simulink model "XMC_FFT2D_HLS_AIE"  (R2021a)
settings: Solver=VariableStepAuto  StartTime=0.0  StopTime=256*256*2  RelTol=1e-3
PreLoadFcn:
  | % display k space image & load arrays for
  | % simulation run
  | MRIDemo_PreloadFcn;
undefined symbols (not defined in the file): gray, S, vsva2197, xcvc1902
libraries: dspxfrm3 x2, dspsrcs4 x2, aieDSP x2, simulink x1, vmcUtilities x1, aieUtilities x1, hlsBasic x1
settings Model: Creator=mmi  LastModifiedBy=abehbood
settings SolverCC: AlgebraicLoopSolver=TrustRegion
settings DataIOCC: ReturnWorkspaceOutputs=off
settings DebuggingCC: SFMachineParentedDataDiag=warning  ArithmeticOperatorsInVariantConditions=warning
settings SFSimCC: SimUseLocalCustomCode=off  CustomCodeUndefinedFunction=UseInterfaceOnly
settings RTWCC: RTWUseLocalCustomCode=off

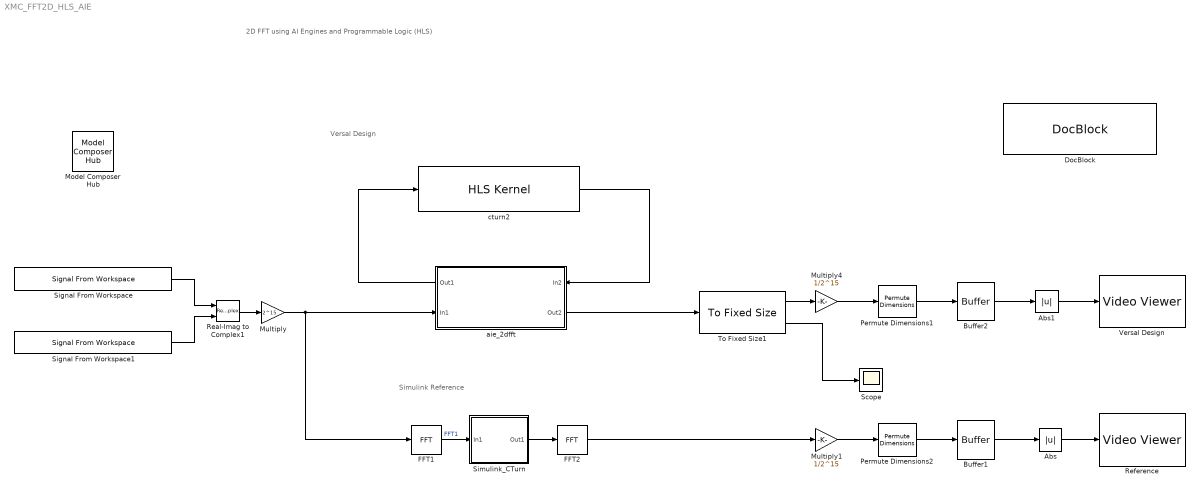
== system XMC_FFT2D_HLS_AIE ==
  note: Versal Design
  note: Simulink Reference
  note: 2D FFT using
      | AI Engines and Programmable Logic (HLS)
  Abs : Abs
  Abs1 : Abs
  Buffer1 : Buffer  N=256  OutputFrames=off
  Buffer2 : Buffer  N=256  OutputFrames=off
  DocBlock : simulink/Model-Wide Utilities/DocBlock  DocumentType=Text  mask(DocBlock){}
      content=|
      | ///////////////////////////////////////////////////////////////////////////
      | // Copyright 2021 Xilinx
      | //
      | // Licensed under the Apache License, Version 2.0 (the "License");
      | // you may not use this file except in compliance with the License.
      | // You may obtain a copy of the License at
      | //
      | // http://www.apache.org/licenses/LICENSE-2.0
      | //
      | // Unless required by applicable law or agreed to in writing, software
      | // distributed under the License is distributed on an "AS IS" BASIS,
      | // WITHOUT WARRANTIES OR CONDITIONS OF ANY KIND, either express or implied.
      | // See the License for the specific language governing permissions and
      | // limitations under the License.
      | ///////////////////////////////////////////////////////////////////////////
      mask Display:
      | xmcDrawBlockIcon();
      | disp(['{\fontsize{10pt}(c) Copyright 2021' ' Xilinx, Inc.}\newline \newline '],'texmode','on');
      | disp('{\fontsize{10pt}Licensed under the Apache License 2.0}','texmode','on');
      | disp('\newline \newline \newline{\fontsize{10pt}Double Click for Copyright Notice}','texmode','on');
  FFT1 : dspxfrm3/FFT  FFTImplementation=Auto  CompMethod=Table lookup  TableOpt=NEW  TableOptActive=Speed  BitRevOrder=off  Normalize=off  InheritFFTLength=on  FFTLength=64  WrapInput=on  roundingMode=Floor  overflowMode=off  firstCoeffDataTypeStr=Inherit: Same word length as input  firstCoeffLastDataTypeStr=Inherit: Same word length as input  prodOutputMode=Binary point scaling  prodOutputWordLength=32  prodOutputFracLength=0  prodOutputDataTypeStr=fixdt(1,32,0)  prodOutputLastDataTypeStr=fixdt(1,32,0)  accumMode=Binary point scaling  accumWordLength=48  accumFracLength=0  accumDataTypeStr=fixdt(1,48,0)  accumLastDataTypeStr=fixdt(1,48,0)  outputMode=Binary point scaling  outputWordLength=16  outputFracLength=0  outputDataTypeStr=fixdt(1,16,0)  outputMin=[]  outputMax=[]  outputLastDataTypeStr=fixdt(1,16,0)
  FFT2 : dspxfrm3/FFT  FFTImplementation=Auto  CompMethod=Table lookup  TableOpt=NEW  TableOptActive=Speed  BitRevOrder=off  Normalize=off  InheritFFTLength=on  FFTLength=64  WrapInput=on  roundingMode=Floor  overflowMode=off  firstCoeffDataTypeStr=Inherit: Same word length as input  firstCoeffLastDataTypeStr=Inherit: Same word length as input  prodOutputMode=Binary point scaling  prodOutputWordLength=32  prodOutputFracLength=0  prodOutputDataTypeStr=fixdt(1,32,0)  prodOutputLastDataTypeStr=fixdt(1,32,0)  accumMode=Binary point scaling  accumWordLength=48  accumFracLength=0  accumDataTypeStr=fixdt(1,48,0)  accumLastDataTypeStr=fixdt(1,48,0)  outputMode=Binary point scaling  outputWordLength=16  outputFracLength=0  outputDataTypeStr=fixdt(1,16,0)  outputMin=[]  outputMax=[]  outputLastDataTypeStr=fixdt(1,16,0)
  Model Composer Hub : vmcUtilities/Model Composer Hub  Tag=genX  CodeGeneration=off  SubsystemName=aie_2dfft  TargetDirectory=./code_fft_graph  ExportType=AI Engines  IpVendor=xilinx.com  IpLibrary=hls  IpVersion=1.0  IpHWLanguage=Verilog  AieCompilerOptions={}  CreateTestbench=on  TestbenchStackSize=10  RunAieSim=on  AieSimTimeout=50000  RunAieSimProfiling=off  LaunchVitisAnalyzer=off  PlotOutput=off  RunX86Sim=off  X86SimTimeout=10  GenHwImage=off  PlatformType=Not Specified  HwSystemType=Baremetal  HwValidationTarget=hw  ProjDevice=xcvc1902-vsva2197-2MP-e-S  ProjDevicePart=xcvc1902-vsva2197-2MP-e-S  SamplePeriod=-1  ClockFrequency=200  DataPathParallelism=1  xilinxfamily=Kintex7  part=xc7k325t  speed=-3  package=fbg676  directory=./netlist  testbench=off  incr_netlist=off  synthesis_tool=Vivado  clock_wrapper=Clock Enables  dbl_ovrd=According to Block Masks  dcm_input_clock_period=10  sysclk_period=10  simulink_period=1  eval_field=0
  Multiply : Gain  Gain=2^15  OutDataTypeStr=int16
  Multiply1 : Gain  Gain=1/2^15  OutDataTypeStr=single
  Multiply4 : Gain  Gain=1/2^15  OutDataTypeStr=single
  Permute Dimensions1 : PermuteDimensions
  Permute Dimensions2 : PermuteDimensions
  Real-Imag to Complex1 : RealImagToComplex
  Reference : VideoViewer  Description=Simulink MRI Display  colormapValue=gray(256)  FigPos=[146 769 633 291]
  Scope : Scope
  Signal From Workspace : dspsrcs4/Signal From Workspace  X=MRIDemo_data_real_channel  Ts=1  nsamps=256  OutputAfterFinalValue=Setting to zero  ignoreOrWarnInputAndFrameLengths=off  OutputFrames=off
  Signal From Workspace1 : dspsrcs4/Signal From Workspace  X=MRIDemo_data_imag_channel  Ts=1  nsamps=256  OutputAfterFinalValue=Setting to zero  ignoreOrWarnInputAndFrameLengths=off  OutputFrames=off
  Simulink_CTurn : Subsystem
  To Fixed Size1 : aieUtilities/To Fixed Size  OutputSize=256  CopyMethod=Buffer samples to form output  HasStatusOutput=off
  Versal Design : VideoViewer  Description=Simulink MRI Display  colormapValue=gray(256)  FigPos=[1240 884 685 270]
  aie_2dfft : Subsystem
      settings: PortSchema="{\"entries\":[{\"content\":{\"sides\":[{\"content\":{\"connectorIds\":[\"Out2\",\"In1\"]},\"type\":\"ConnectorPlacement.EquallySpacedRectSide\",\"uuid\":\"79f05cc3-f11a-4cde-8fa1-dcc9430b22c8\"},{\"content\":{\"connectorIds\":[\"In2\",\"Out1\"],\"side\":\"RIGHT\"},\"type\":\"ConnectorPlacement.EquallySpacedRectSide\",\"uuid\":\"dca5e86a-9095-4cba-ba8f-7e749e0dbd7e\"},{\"content\":{\"connectorIds\":[],\"side\":\"TOP\"},\"type\":\"ConnectorPlacement.EquallySpacedRectSide\",\"uuid\":\"3830c194-8485-43cd-afe1-c92005d5a3f9\"}]},\"type\":\"ConnectorPlacement.EquallySpacedConnector\",\"uuid\":\"40ec3e32-3e8f-4730-8170-0d4e5db1f984\"}],\"packageUris\":[\"http://schema.mathworks.com/mf0/Connector/19700101\"],\"version\":\"1.0\"}"
  cturn2 : hlsBasic/HLS Kernel  PortNames={}  PortSerializedTypes={}  FunctionTemplateParamNames={}  FunctionTemplateParamKinds={}  FunctionTemplateParamTypes={}  FunctionTemplateParamValues={}  PortSynchronicities={'auto'; 'auto'}  PortSignalSizes={0.000000000000000000e+00; 2.560000000000000000e+02}  FunctionTemplateParams={}  FunctionTemplateParamsEnables={}  FunctionTemplateParamsVisible=off  FunctionDeclTypeOptions=C[1 1]@t7@<empty>  PortAttributesTable={ 'Input', 'vin', 'hls::stream< std::complex< int16 >, 0 > &', '', ''; 'Output', 'vout', 'hls::stream< std::complex< int16 >, 0 > &', '', '256' }  PortAttributesEnablement={'off', 'off', 'off', 'off', 'off';'off', 'off', 'off', 'off', 'on'}  SampleTime=-1  PortDirectionTable={ 'vin', 'hls::stream< std::complex< int16 >, 0 > &', 'Input'; 'vout', 'hls::stream< std::complex< int16 >, 0 > &', 'Output' }  PortDirectionTabVisible=on  ArgDirections={1.000000000000000000e+00; 2.000000000000000000e+00}  FunctionIndex=1  FormalArgDecls={'hls::stream< std::complex< int16 >, 0 > & vin', 'hls::stream< std::complex< int16 >, 0 > & vout'}  SimLibPath=''  FunctionTabVisible=on  FunctionDescription=void cturn2(hls::stream< std::complex< int16 >, 0 > & vin, hls::stream< std::complex< int16 >, 0 > & vout)  KernelHeaderFile=./src/cturn2.h  KernelFunction=cturn2  KernelFunctionSelect=<empty>  KernelSourceFile=./src/cturn2.cpp  KernelSearchPaths={}  PreProcOptions={}  blockJsonConstraints=[]  deprecateConstraints=0
  wires:
  Signal From Workspace/1 -> Real-Imag to Complex1/1
  Signal From Workspace1/1 -> Real-Imag to Complex1/2
  FFT2/1 -> Multiply1/1
  Buffer1/1 -> Abs/1
  Permute Dimensions2/1 -> Buffer1/1
  Abs/1 -> Reference/1
  FFT1/1 -> Simulink_CTurn/1(In1)  "FFT1"
  Simulink_CTurn/1(Out1) -> FFT2/1
  Multiply/1 -> FFT1/1, aie_2dfft/1(In1)
  Multiply1/1 -> Permute Dimensions2/1
  Real-Imag to Complex1/1 -> Multiply/1
  Buffer2/1 -> Abs1/1
  Abs1/1 -> Versal Design/1
  To Fixed Size1/1 -> Multiply4/1
  Permute Dimensions1/1 -> Buffer2/1
  aie_2dfft/1(Out2) -> To Fixed Size1/1
  Multiply4/1 -> Permute Dimensions1/1
  aie_2dfft/2(Out1) -> cturn2/1
  cturn2/1 -> aie_2dfft/2(In2)
  To Fixed Size1/2 -> Scope/1

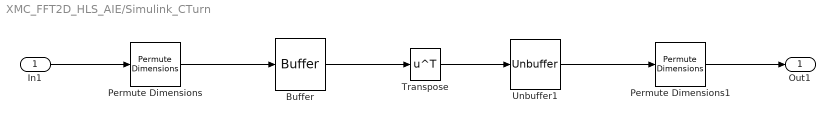
== system XMC_FFT2D_HLS_AIE/Simulink_CTurn ==
  In1 : Inport
  Buffer : Buffer  N=256  OutputFrames=off
  Permute Dimensions : PermuteDimensions
  Permute Dimensions1 : PermuteDimensions
  Transpose : Math  Operator=transpose  SignedPower=on  SaturateOnIntegerOverflow=on
  Unbuffer1 : Unbuffer
  Out1 : Outport  VectorParamsAs1DForOutWhenUnconnected=off
  wires:
  Permute Dimensions/1 -> Buffer/1
  Transpose/1 -> Unbuffer1/1
  Buffer/1 -> Transpose/1
  In1/1 -> Permute Dimensions/1
  Unbuffer1/1 -> Permute Dimensions1/1
  Permute Dimensions1/1 -> Out1/1

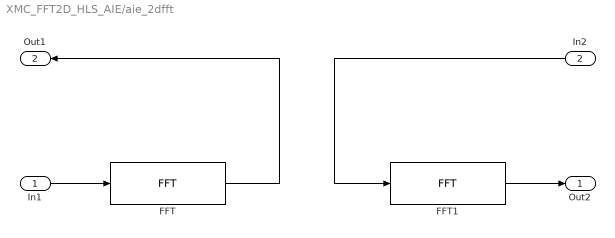
== system XMC_FFT2D_HLS_AIE/aie_2dfft ==
  In1 : Inport
  In2 : Inport  Port=2
  FFT : aieDSP/FFT  data_type=cint16  point_size=256  input_window_size=256  shift_val=0  input_sampling_rate=200  use_casc_length=on  casc_length=1  spec=meta_data_hl_fft.json
  FFT1 : aieDSP/FFT  data_type=cint16  point_size=256  input_window_size=256  shift_val=0  input_sampling_rate=200  use_casc_length=on  casc_length=1  spec=meta_data_hl_fft.json
  Out2 : Outport
  Out1 : Outport  Port=2
  wires:
  FFT/1 -> Out1/1
  FFT1/1 -> Out2/1
  In1/1 -> FFT/1
  In2/1 -> FFT1/1
